simulink model "simulink1_1c"  (R2025b)
settings: Solver=VariableStepAuto  StartTime=0.0  StopTime=1  RelTol=1e-3
settings Model: Creator=getrj  LastModifiedBy=owenm

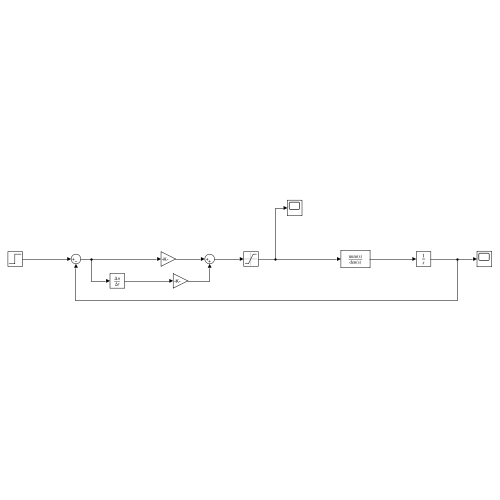
[thumbnail: Simulink's stored preview of the top-level diagram]
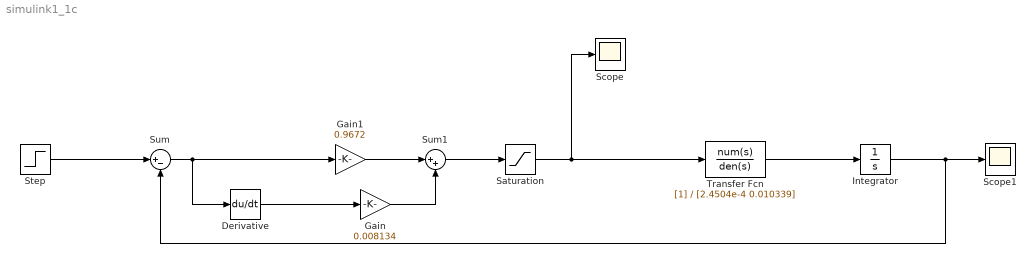
== system simulink1_1c ==
  Derivative : Derivative
  Gain : Gain  Gain=0.008134
  Gain1 : Gain  Gain=0.9672
  Integrator : Integrator
  Saturation : Saturate  UpperLimit=10  LowerLimit=-10
  Scope : Scope
      settings: ActiveDisplayYMinimum=-1.0129203936463997  ActiveDisplayYMaximum=1.1872133770718221
  Scope1 : Scope
      settings: ActiveDisplayYMinimum=-0.0740190078435875  ActiveDisplayYMaximum=1.0869922838518802
  Step : Step  Time=0  SampleTime=0
  Sum : Sum  Inputs=|+-
  Sum1 : Sum  Inputs=|++
  Transfer Fcn : TransferFcn  Denominator=[2.4504e-4 0.010339]
  wires:
  Step/1 -> Sum/1
  Sum/1 -> Derivative/1, Gain1/1
  Gain1/1 -> Sum1/1
  Gain/1 -> Sum1/2
  Sum1/1 -> Saturation/1
  Saturation/1 -> Transfer Fcn/1, Scope/1
  Transfer Fcn/1 -> Integrator/1
  Integrator/1 -> Sum/2, Scope1/1
  Derivative/1 -> Gain/1
